simulink model "train"  (R2013a)
settings: Solver=ode45  StartTime=0.0  StopTime=time  RelTol=1e-3
values from neighbouring files (symbols this model uses):
  adj = 2    [proj.m]
  lqrsat = 200    [proj.m]
  noisePower = 1e3    (= 1000)    [proj.m]
  seed = floor(init*1000) + 7    [proj.m]
  thres = pi/3    (= 1.0471975512)    [proj.m]
  vsat = 50    [proj.m]
undefined symbols (not defined in the file or in its folder): init
libraries: simulink x1
settings Model: Creator=dello  LastModifiedBy=dello

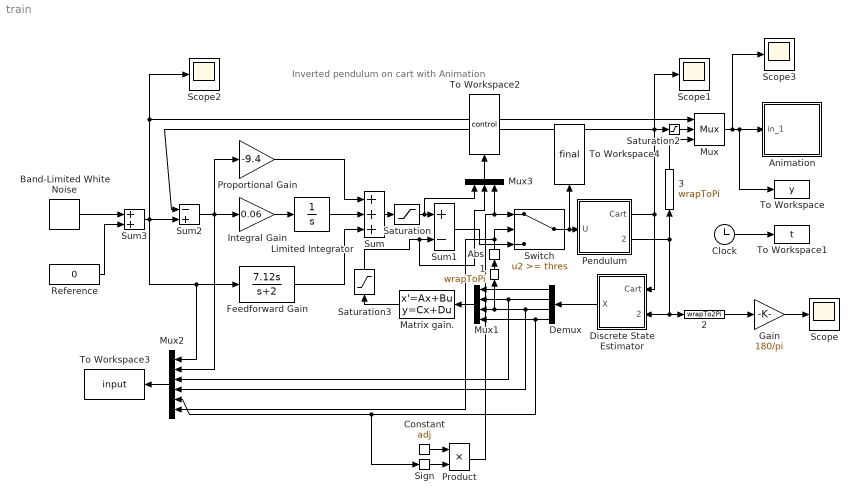
== system train ==
  note: Inverted pendulum on cart with Animation
  " 1" : MATLABFcn  MATLABFcn=wrapToPi
  " 2" : MATLABFcn  MATLABFcn=wrapTo2Pi
  " 3" : MATLABFcn  MATLABFcn=wrapToPi
  Abs : Abs
  Animation : Subsystem  mask(Pendulum plot){RefBlock=Reference}
      mask prompts: RefBlock "DC reference signal block name:"
      mask help: Pendulum plot
      mask Help: Pendulum animation function using Handle graphics.
      mask Display: plot([-10 10],[0 0],[-2 -2 2 2],[0 1 1 0],[0 3],[1 5])
  Band-Limited White Noise : simulink/Sources/Band-Limited White Noise  Cov=[noisePower]  Ts=10  seed=[seed]
  Clock : Clock
  Constant : Constant  Value=adj
  Demux : Demux
  Discrete State Estimator : Subsystem  mask(Pendulum Discrete state estimator){Ts=0.02}
      mask prompts: Ts "Sample time"
      mask help: Pendulum discrete state estimator
      mask Help: The states of the pendulum and cart system are the pendulum angle and angular velocity and cart position and velocity.  Since the sensors output the pendulum angle and cart position, this state estimator just does a one step difference calculation to get the velocities.
  Feedforward Gain : TransferFcn  Numerator=[7.12 0]  Denominator=[1 2]
  Gain : Gain  Gain=180/pi
  Integral Gain : Gain  Gain=0.06  SaturateOnIntegerOverflow=on  OutDataTypeStr=Inherit: Same as input  ParamDataTypeStr=Inherit: Same as input
  Limited Integrator : Integrator  LimitOutput=on  UpperSaturationLimit=5  LowerSaturationLimit=-5
  Matrix gain. : StateSpace  A=[]  B=[]  C=[]  D=K  mask(Matrix gain){K=[0 -18 -166.5 -15.2]}
      mask prompts: K "Gain matrix:"
      mask help: Matrix Gain:
      mask Help: Multiplies input vector by entered matrix to produce output vector.
      mask Display: disp('LQR')
  Mux : Mux  Inputs=3
  Mux1 : Mux
  Mux2 : Mux  Inputs=6
  Mux3 : Mux  Inputs=3
  Pendulum : Subsystem  mask(Inverted pendulum on cart){Mcart=0.455, m=0.21, l=0.61/2, g=9.8}
      mask prompts: Mcart "Mass of cart (kg):"; m "Mass of pendulum (kg):"; l "Distance to pendulum center of mass(m):"; g "Acceleration of gravity (m/s^2):"
      mask help: Unmask and double-click to see dynamics
      mask Help: Nonlinear dynamics of inverted pendulum on cart.
  Product : Product
  Proportional Gain : Gain  Gain=-9.4  SaturateOnIntegerOverflow=on  OutDataTypeStr=Inherit: Same as input  ParamDataTypeStr=Inherit: Same as input
  Reference : Constant  Value=0
  Saturation : Saturate  UpperLimit=vsat  LowerLimit=-vsat
  Saturation2 : Saturate  UpperLimit=10  LowerLimit=-10
  Saturation3 : Saturate  UpperLimit=lqrsat  LowerLimit=-lqrsat
  Scope{,1..3} (4 alike) : Scope
      Scope settings: TimeRange=50  YMin=3.105  YMax=3.18
      Scope2 settings: SaveName=ScopeData2
      Scope3 settings: SaveName=ScopeData3
  Sign : Signum
  Sum : Sum  Inputs=+++  SaturateOnIntegerOverflow=on  InputSameDT=on  OutDataTypeStr=Inherit: Same as first input
  Sum1 : Sum  Inputs=+-  SaturateOnIntegerOverflow=on  InputSameDT=on  OutDataTypeStr=Inherit: Same as first input
  Sum2 : Sum  Inputs=-+  SaturateOnIntegerOverflow=on  InputSameDT=on  OutDataTypeStr=Inherit: Same as first input
  Sum3 : Sum  SaturateOnIntegerOverflow=on  InputSameDT=on  OutDataTypeStr=Inherit: Same as first input
  Switch : Switch  Threshold=thres
  To Workspace : ToWorkspace  VariableName=y  SampleTime=0.1
  To Workspace1 : ToWorkspace  VariableName=t  SampleTime=0.1
  To Workspace2 : ToWorkspace  VariableName=control  SampleTime=-1
  To Workspace3 : ToWorkspace  VariableName=input  SampleTime=-1
  To Workspace4 : ToWorkspace  VariableName=final  SampleTime=-1
  wires:
  Sum2/1 -> Mux2/2, Proportional Gain/1, Integral Gain/1
  Mux/1 -> Scope3/1, To Workspace/1, Animation/1(in_1)
  Sum3/1 -> Mux2/1, Feedforward Gain/1, Sum2/2, Scope2/1, Mux/1
  Integral Gain/1 -> Limited Integrator/1
  Sum/1 -> Saturation/1
  Proportional Gain/1 -> Sum/1
  Feedforward Gain/1 -> Sum/3
  Reference/1 -> Sum3/2
  Band-Limited White Noise/1 -> Sum3/1
  Limited Integrator/1 -> Sum/2
  Pendulum/1(Cart) -> Sum2/1, Saturation2/1, Scope1/1, Discrete State Estimator/1(Cart)
  Clock/1 -> To Workspace1/1
  Saturation/1 -> Mux3/1, Sum1/1
  Mux1/1 -> Matrix gain./1
  Discrete State Estimator/1(X) -> Demux/1
  Demux/1 -> Mux1/1
  Demux/2 -> Mux2/3, Mux1/2
  Demux/3 -> Mux2/4, " 1"/1, Mux1/3
  Demux/4 -> Sign/1, Mux2/5, Mux1/4
  " 2"/1 -> Gain/1
  " 3"/1 -> Mux/3
  Saturation2/1 -> Mux/2
  Matrix gain./1 -> Saturation3/1
  Saturation3/1 -> Mux3/2, Sum1/2
  Mux2/1 -> To Workspace3/1
  Switch/1 -> Pendulum/1(U), To Workspace4/1
  Sum1/1 -> Switch/3
  " 1"/1 -> Abs/1
  Constant/1 -> Product/1
  Sign/1 -> Product/2
  Product/1 -> Mux3/3, Switch/1
  Abs/1 -> Mux2/6, Switch/2
  Gain/1 -> Scope/1
  Pendulum/2(Pendulum) -> Discrete State Estimator/2(Pendulum), " 2"/1, " 3"/1
  Mux3/1 -> To Workspace2/1

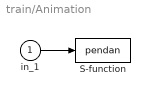
== system train/Animation ==
  in_1 : Inport
  S-function : S-Function  FunctionName=pendan  Parameters=RefBlock  EnableBusSupport=off
      settings: DeleteFcn=pendan([],[],[],'DeleteBlock');
  wires:
  in_1/1 -> S-function/1

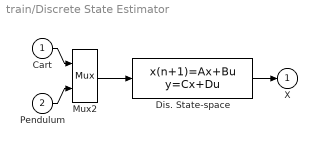
== system train/Discrete State Estimator ==
  Cart : Inport
  Pendulum : Inport  Port=2
  Dis. State-space : DiscreteStateSpace  A=zeros(2)  B=-eye(2)/Ts  C=[0 0; 1 0; 0 0; 0 1]  D=[1 0; 1/Ts 0; 0 1; 0 1/Ts]  SampleTime=Ts
  Mux2 : Mux  Inputs=2
  X : Outport  InitialOutput=0
  wires:
  Pendulum/1 -> Mux2/2
  Dis. State-space/1 -> X/1
  Cart/1 -> Mux2/1
  Mux2/1 -> Dis. State-space/1

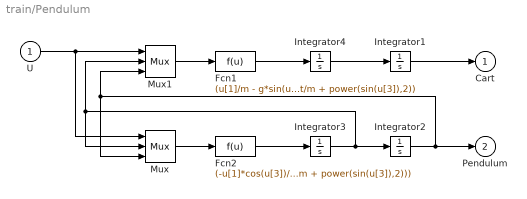
== system train/Pendulum ==
  U : Inport
  Fcn1 : Fcn  Expr=(u[1]/m - g*sin(u[3])*cos(u[3]) + l*power(u[2],2)*sin(u[3]))/(Mcart/m + power(sin(u[3]),2))
  Fcn2 : Fcn  Expr=(-u[1]*cos(u[3])/m + (Mcart+m)*g*sin(u[3])/m - l*power(u[2],2)*sin(u[3])*cos(u[3]))/(l*(Mcart/m + power(sin(u[3]),2)))
  Integrator1 : Integrator
  Integrator2 : Integrator  InitialCondition=init
  Integrator3 : Integrator
  Integrator4 : Integrator
  Mux : Mux  Inputs=3
  Mux1 : Mux  Inputs=3
  Cart : Outport  InitialOutput=0
  Pendulum : Outport  Port=2  InitialOutput=0
  wires:
  Integrator1/1 -> Cart/1
  Fcn2/1 -> Integrator3/1
  Mux/1 -> Fcn2/1
  Mux1/1 -> Fcn1/1
  Fcn1/1 -> Integrator4/1
  Integrator4/1 -> Integrator1/1
  U/1 -> Mux1/1, Mux/1
  Integrator3/1 -> Integrator2/1, Mux1/2, Mux/2
  Integrator2/1 -> Pendulum/1, Mux1/3, Mux/3
